simulink model "Senorless"  (R2023a)
settings: Solver=FixedStepDiscrete  StartTime=0.0  StopTime=2  FixedStep=1/FOC_FRQ  RelTol=1e-3
values from neighbouring files (symbols this model uses):
  ADC_REF = 3.6    [Senorless.sldd]
  ADC_SAMPLE_MAX = 32767.0    [Senorless.sldd]
  AMP_GAIN = 32.0    [Senorless.sldd]
  CURR_INPUT = 3276.0    [Senorless.sldd]
  CURR_KI = 380.0    [Senorless.sldd]
  CURR_KP = 0.04    [Senorless.sldd]
  CURR_LIMIT = 1.1    [Senorless.sldd]
  CURR_OVER = 34.0    [Senorless.sldd]
  CURR_POINT_GAIN = 7.0    [Senorless.sldd]
  CURR_STEP = 32760.0    [Senorless.sldd]
  CURR_UNDER = 0.03    [Senorless.sldd]
  CURR_WIDTH = 250.0    [Senorless.sldd]
  FOC_FRQ = 36000.0    [Senorless.sldd]
  GAMMA = 32767.0    [Senorless.sldd]
  HFI_ID = 2.125    [Senorless.sldd]
  IMAX = 34.0    [Senorless.sldd]
  LPF_FRQ = 300.0    [Senorless.sldd]
  MOTOR_DAMPER = 8.3E-7    [Senorless.sldd]
  MOTOR_FLUX = 0.0012713112    [Senorless.sldd]
  MOTOR_INERTIA = 1.02E-6    [Senorless.sldd]
  MOTOR_LS = 1.8E-5    [Senorless.sldd]
  MOTOR_PN = 7.0    [Senorless.sldd]
  MOTOR_RS = 0.065    [Senorless.sldd]
  NS_COMP_UD = 0.531    [Senorless.sldd]
  PLL_LIMIT = 0.95    [Senorless.sldd]
  PLL_WIDTH = 500.0    [Senorless.sldd]
  PWM_FRQ = 96000000.0    [Senorless.sldd]
  RS_HUNT = 0.002    [Senorless.sldd]
  SMOK_FRQ = 1200.0    [Senorless.sldd]
  SPD_LIMIT = 0.8    [Senorless.sldd]
  SPD_LPF_LEVEL = 15.0    [Senorless.sldd]
  SPD_MAX = 8100.0    [Senorless.sldd]
  SPD_MIN = -8100.0    [Senorless.sldd]
  SPD_REDUCE = 380.0    [Senorless.sldd]
  SPD_STEP = 3.0    [Senorless.sldd]
  SPD_WIDTH = 10.0    [Senorless.sldd]
  TS_POINT_GAIN = 10.0    [Senorless.sldd]
  UDC = 17.0    [Senorless.sldd]
  UDC_GAIN = 21.0    [Senorless.sldd]
  UDC_POINT_GAIN = 10.0    [Senorless.sldd]
undefined symbols (not defined in the file or in its folder): curr_q_ki, curr_q_kp, DiscIntNeverNeededParam, magnitude, PLL_LPF_LEVEL, Udc
libraries: simulink x20, slpidlib x5, mcbcontrolslib x4, mcbplantlib x1, autolibpmsminterior x1, autolibpmsmexterior x1, spspowerguiLib x1
(part 6 of 7)

== system Senorless/FOC_PointModel/Observers/SMO/SMO_LPF1 ==
  note: y(n)=ax(n)+(1−a)y(n−1)
  note: a =(ω c​ T s​ )/(1+ω c​ T s​ )
  input : Inport
  Constant5 : Constant  Value=32767  OutDataTypeStr=int16
  Data Store Read1 : DataStoreRead  DataStoreName=LPF_FRQ_Point  IndexOptions=Index vector (dialog)  Indices=1  OutputSizes=1
  Data Store Read7 : DataStoreRead  DataStoreName=LPF_FRQ_Point  IndexOptions=Index vector (dialog)  Indices=1  OutputSizes=1
  Product1 : Product  OutDataTypeStr=int32  RndMeth=Zero
  Product10 : Product  OutDataTypeStr=int32
  Product11 : Product  OutDataTypeStr=int32  RndMeth=Zero
  Shift Arithmetic2 : ArithShift  BitShiftNumber=15
  Shift Arithmetic3 : ArithShift  BitShiftNumber=15
  Shift Arithmetic4 : ArithShift  BitShiftNumber=4
  Sum1 : Sum  Inputs=-+  OutDataTypeStr=int32  RndMeth=Zero
  Sum10 : Sum  Inputs=-+  OutDataTypeStr=int16  RndMeth=Zero
  Sum11 : Sum  OutDataTypeStr=int32  RndMeth=Zero
  Sum2 : Sum  OutDataTypeStr=int32  RndMeth=Zero
  Unit Delay1 : UnitDelay  SampleTime=-1  HasFrameUpgradeWarning=on
  Unit Delay9 : UnitDelay  SampleTime=-1  HasFrameUpgradeWarning=on
  input1 : InportShadow
  output : Outport
  wires:
  Product10/1 -> Shift Arithmetic3/1
  Product11/1 -> Shift Arithmetic2/1
  Unit Delay9/1 -> Product10/2
  Sum10/1 -> Product10/1
  input/1 -> Product11/1
  Data Store Read7/1 -> Sum10/1, Product11/2
  Sum11/1 -> Unit Delay9/1
  Shift Arithmetic2/1 -> Sum11/1
  Shift Arithmetic3/1 -> Sum11/2
  input1/1 -> Sum1/2
  Unit Delay1/1 -> Sum2/1, Sum1/1
  Sum2/1 -> output/1, Unit Delay1/1
  Sum1/1 -> Product1/1
  Data Store Read1/1 -> Product1/2
  Product1/1 -> Shift Arithmetic4/1
  Shift Arithmetic4/1 -> Sum2/2
  Constant5/1 -> Sum10/2

== system Senorless/FOC_PointModel/Observers/SMO/SMO_LPF2 ==
  note: a =(ω c​ T s​ )/(1+ω c​ T s​ )
  note: y(n)=ax(n)+(1−a)y(n−1)
  input : Inport
  Constant5 : Constant  Value=32767  OutDataTypeStr=int16
  Data Store Read1 : DataStoreRead  DataStoreName=LPF_FRQ_Point  IndexOptions=Index vector (dialog)  Indices=1  OutputSizes=1
  Data Store Read7 : DataStoreRead  DataStoreName=LPF_FRQ_Point  IndexOptions=Index vector (dialog)  Indices=1  OutputSizes=1
  Product1 : Product  OutDataTypeStr=int32  RndMeth=Zero
  Product10 : Product  OutDataTypeStr=int32
  Product11 : Product  OutDataTypeStr=int32  RndMeth=Zero
  Shift Arithmetic2 : ArithShift  BitShiftNumber=15
  Shift Arithmetic3 : ArithShift  BitShiftNumber=15
  Shift Arithmetic4 : ArithShift  BitShiftNumber=4
  Sum1 : Sum  Inputs=-+  OutDataTypeStr=int32  RndMeth=Zero
  Sum10 : Sum  Inputs=-+  OutDataTypeStr=int16  RndMeth=Zero
  Sum11 : Sum  OutDataTypeStr=int32  RndMeth=Zero
  Sum2 : Sum  OutDataTypeStr=int32  RndMeth=Zero
  Unit Delay1 : UnitDelay  SampleTime=-1  HasFrameUpgradeWarning=on
  Unit Delay9 : UnitDelay  SampleTime=-1  HasFrameUpgradeWarning=on
  input1 : InportShadow
  output : Outport
  wires:
  Shift Arithmetic4/1 -> Sum2/2
  Product1/1 -> Shift Arithmetic4/1
  Data Store Read1/1 -> Product1/2
  Sum1/1 -> Product1/1
  Sum2/1 -> output/1, Unit Delay1/1
  Unit Delay1/1 -> Sum1/1, Sum2/1
  input1/1 -> Sum1/2
  Shift Arithmetic3/1 -> Sum11/2
  Shift Arithmetic2/1 -> Sum11/1
  Data Store Read7/1 -> Product11/2, Sum10/1
  Constant5/1 -> Sum10/2
  input/1 -> Product11/1
  Sum10/1 -> Product10/1
  Unit Delay9/1 -> Product10/2
  Product11/1 -> Shift Arithmetic2/1
  Product10/1 -> Shift Arithmetic3/1
  Sum11/1 -> Unit Delay9/1

== system Senorless/FOC_PointModel/Observers/SMO/SMO_LPF4 ==
  note: a =(ω c​ T s​ )/(1+ω c​ T s​ )
  note: y(n)=ax(n)+(1−a)y(n−1)
  input : Inport
  Constant5 : Constant  OutDataTypeStr=int16
  Data Store Read7 : DataStoreRead  DataStoreName=LPF_FRQ_Point  IndexOptions=Index vector (dialog)  Indices=1  OutputSizes=1
  Data Type Conversion6 : DataTypeConversion  OutDataTypeStr=int16  SaturateOnIntegerOverflow=off
  Product10 : Product  OutDataTypeStr=int32
  Product11 : Product  OutDataTypeStr=int32  RndMeth=Zero
  Shift Arithmetic1 : ArithShift  BitShiftNumber=-4
  Shift Arithmetic9 : ArithShift  BitShiftNumber=4
  Sum10 : Sum  Inputs=-+
  Sum11 : Sum  OutDataTypeStr=int32  RndMeth=Zero
  Unit Delay9 : UnitDelay  SampleTime=-1  HasFrameUpgradeWarning=on
  output : Outport
  wires:
  Constant5/1 -> Shift Arithmetic1/1
  Sum11/1 -> Shift Arithmetic9/1
  Data Type Conversion6/1 -> output/1, Unit Delay9/1
  Shift Arithmetic9/1 -> Data Type Conversion6/1
  Data Store Read7/1 -> Product11/2, Sum10/1
  Shift Arithmetic1/1 -> Sum10/2
  input/1 -> Product11/1
  Sum10/1 -> Product10/1
  Unit Delay9/1 -> Product10/2
  Product11/1 -> Sum11/1
  Product10/1 -> Sum11/2

== system Senorless/FOC_PointModel/Observers/SMO/SMO_LPF5 ==
  note: y(n)=ax(n)+(1−a)y(n−1)
  note: a =(ω c​ T s​ )/(1+ω c​ T s​ )
  input : Inport
  Constant5 : Constant  OutDataTypeStr=int16
  Data Store Read7 : DataStoreRead  DataStoreName=LPF_FRQ_Point  IndexOptions=Index vector (dialog)  Indices=1  OutputSizes=1
  Data Type Conversion6 : DataTypeConversion  OutDataTypeStr=int16  SaturateOnIntegerOverflow=off
  Product10 : Product  OutDataTypeStr=int32
  Product11 : Product  OutDataTypeStr=int32  RndMeth=Zero
  Shift Arithmetic1 : ArithShift  BitShiftNumber=-4
  Shift Arithmetic9 : ArithShift  BitShiftNumber=4
  Sum10 : Sum  Inputs=-+
  Sum11 : Sum  OutDataTypeStr=int32  RndMeth=Zero
  Unit Delay9 : UnitDelay  SampleTime=-1  HasFrameUpgradeWarning=on
  output : Outport
  wires:
  Product10/1 -> Sum11/2
  Product11/1 -> Sum11/1
  Unit Delay9/1 -> Product10/2
  Sum10/1 -> Product10/1
  input/1 -> Product11/1
  Shift Arithmetic1/1 -> Sum10/2
  Data Store Read7/1 -> Sum10/1, Product11/2
  Shift Arithmetic9/1 -> Data Type Conversion6/1
  Data Type Conversion6/1 -> Unit Delay9/1, output/1
  Sum11/1 -> Shift Arithmetic9/1
  Constant5/1 -> Shift Arithmetic1/1

== system Senorless/FOC_PointModel/Observers/SMO/Subsystem ==
  ialpha_err : Inport
  ialpha_hat : Inport  Port=2
  ibeta_hat : Inport  Port=3
  ibeta_err : Inport  Port=4
  Constant : Constant  Value=MOTOR_RS
  Display : Display
  Display1 : Display
  Divide : Product  Inputs=*/
  Gain4 : Gain  Gain=1/MOTOR_LS/FOC_FRQ
  Product : Product
  Product1 : Product
  Scope : Scope
  Scope1 : Scope  NumInputPorts=2
  Scope2 : Scope
  Scope3 : Scope  NumInputPorts=2
  Sum : Sum  Inputs=|++
  Sum2 : Sum
  Unit Delay : UnitDelay  SampleTime=-1  HasFrameUpgradeWarning=on
  Output : Outport
  wires:
  ibeta_hat/1 -> Product1/2
  ialpha_hat/1 -> Scope3/2, Product/2
  Product/1 -> Scope1/1, Sum2/1
  Constant/1 -> Divide/1, Display/1
  Divide/1 -> Display1/1
  Product1/1 -> Scope1/2, Sum2/2
  ialpha_err/1 -> Scope3/1, Product/1
  ibeta_err/1 -> Product1/1
  Gain4/1 -> Sum/1
  Sum/1 -> Unit Delay/1, Output/1, Scope2/1, Divide/2
  Unit Delay/1 -> Sum/2
  Sum2/1 -> Scope/1, Gain4/1

== system Senorless/FOC_PointModel/Observers/滤波器/LPF ==
  note: a =(ω c​ T s​ )/(1+ω c​ T s​ )
  note: y(n)=ax(n)+(1−a)y(n−1)
  input : Inport
  Constant1 : Constant  Value=8  OutDataTypeStr=int16
  Constant5 : Constant  OutDataTypeStr=int16
  Product10 : Product  OutDataTypeStr=int32
  Product11 : Product  OutDataTypeStr=int32  RndMeth=Zero
  Saturation : Saturate  UpperLimit=15  LowerLimit=0  RndMeth=Zero
  Shift Arithmetic1 : ArithShift  BitShiftNumber=-4
  Shift Arithmetic9 : ArithShift  BitShiftNumber=4
  Sum10 : Sum  Inputs=-+
  Sum11 : Sum  OutDataTypeStr=int32  RndMeth=Zero
  Unit Delay9 : UnitDelay  SampleTime=-1  HasFrameUpgradeWarning=on
  output : Outport
  wires:
  Constant1/1 -> Saturation/1
  Constant5/1 -> Shift Arithmetic1/1
  Sum11/1 -> Shift Arithmetic9/1
  Shift Arithmetic9/1 -> output/1, Unit Delay9/1
  Shift Arithmetic1/1 -> Sum10/2
  Sum10/1 -> Product10/1
  Product11/1 -> Sum11/1
  Product10/1 -> Sum11/2
  Unit Delay9/1 -> Product11/1
  input/1 -> Product10/2
  Saturation/1 -> Sum10/1, Product11/2

== system Senorless/FOC_PointModel/Observers/滤波器/积分器4 ==
  input : Inport
  Constant : Constant  OutDataTypeStr=int16
  Data Store Read1 : DataStoreRead  DataStoreName=Ts_Point  IndexOptions=Index vector (dialog)  Indices=1  OutputSizes=1
  Data Type Conversion3 : DataTypeConversion  Commented=on  OutDataTypeStr=int16  SaturateOnIntegerOverflow=off
  Divide : Product  Commented=on  Inputs=*/  OutDataTypeStr=int32  RndMeth=Zero
  Product1 : Product  OutDataTypeStr=int32  RndMeth=Zero
  Product2 : Product  OutDataTypeStr=int32  RndMeth=Zero
  Shift Arithmetic : ArithShift  BitShiftNumberSource=Input port  BitShiftNumber=8  BitShiftDirection=Right
      settings: InputPortMap=u0,p1
  Sum : Sum  Inputs=|++  OutDataTypeStr=int32  RndMeth=Zero
  Ts适当放大的缩小系数， 详见初始化模块 : ArithShift  Commented=on  BitShiftNumber=TS_POINT_GAIN  DiagnosticForOORShift=Error
  Unit Delay : UnitDelay  SampleTime=-1  HasFrameUpgradeWarning=on
  周期定点化适当放大2^n : Constant  Value=TS_POINT_GAIN
  积分器运行频率 : Constant  Commented=on  Value=FOC_FRQ
  这个是缩小周期增益的 : ArithShift  BitShiftNumber=15  DiagnosticForOORShift=Error
  output : Outport
  wires:
  这个是缩小周期增益的/1 -> output/1
  Product2/1 -> Product1/2
  积分器运行频率/1 -> Data Type Conversion3/1
  Data Type Conversion3/1 -> Divide/2
  周期定点化适当放大2^n/1 -> Shift Arithmetic/2
  Sum/1 -> Unit Delay/1, 这个是缩小周期增益的/1
  Unit Delay/1 -> Sum/2
  input/1 -> Shift Arithmetic/1
  Shift Arithmetic/1 -> Product2/2
  Data Store Read1/1 -> Product2/1
  Constant/1 -> Product1/1
  Product1/1 -> Sum/1

== system Senorless/FOC_PointModel/Observers/滤波器/积分器5 ==
  input : Inport
  Constant : Constant  OutDataTypeStr=int16
  Data Store Read1 : DataStoreRead  DataStoreName=Ts_Point  IndexOptions=Index vector (dialog)  Indices=1  OutputSizes=1
  Data Type Conversion3 : DataTypeConversion  Commented=on  OutDataTypeStr=int16  SaturateOnIntegerOverflow=off
  Divide : Product  Commented=on  Inputs=*/  OutDataTypeStr=int32  RndMeth=Zero
  Product1 : Product  OutDataTypeStr=int32  RndMeth=Zero
  Product2 : Product  OutDataTypeStr=int32  RndMeth=Zero
  Shift Arithmetic : ArithShift  BitShiftNumberSource=Input port  BitShiftNumber=8  BitShiftDirection=Right
      settings: InputPortMap=u0,p1
  Sum : Sum  Inputs=|++  OutDataTypeStr=int32  RndMeth=Zero
  Ts适当放大的缩小系数， 详见初始化模块 : ArithShift  Commented=on  BitShiftNumber=TS_POINT_GAIN  DiagnosticForOORShift=Error
  Unit Delay : UnitDelay  SampleTime=-1  HasFrameUpgradeWarning=on
  周期定点化适当放大2^n : Constant  Value=TS_POINT_GAIN
  积分器运行频率 : Constant  Commented=on  Value=FOC_FRQ
  这个是缩小周期增益的 : ArithShift  BitShiftNumber=15  DiagnosticForOORShift=Error
  output : Outport
  wires:
  这个是缩小周期增益的/1 -> output/1
  Product2/1 -> Product1/2
  积分器运行频率/1 -> Data Type Conversion3/1
  Data Type Conversion3/1 -> Divide/2
  周期定点化适当放大2^n/1 -> Shift Arithmetic/2
  Sum/1 -> Unit Delay/1, 这个是缩小周期增益的/1
  Unit Delay/1 -> Sum/2
  input/1 -> Shift Arithmetic/1
  Shift Arithmetic/1 -> Product2/2
  Data Store Read1/1 -> Product2/1
  Constant/1 -> Product1/1
  Product1/1 -> Sum/1

== system Senorless/FOC_PointModel/Observers/纯浮点NFO/LPF ==
  note: a =(ω c​ T s​ )/(1+ω c​ T s​ )
  note: y(n)=ax(n)+(1−a)y(n−1)
  input : Inport
  Constant1 : Constant  Value=SPD_LPF_LEVEL  OutDataTypeStr=int16
  Constant5 : Constant  OutDataTypeStr=int16
  Product10 : Product  OutDataTypeStr=int32
  Product11 : Product  OutDataTypeStr=int32  RndMeth=Zero
  Saturation : Saturate  UpperLimit=15  LowerLimit=0  RndMeth=Zero
  Shift Arithmetic1 : ArithShift  BitShiftNumber=-4
  Shift Arithmetic9 : ArithShift  BitShiftNumber=4
  Sum10 : Sum  Inputs=-+
  Sum11 : Sum  OutDataTypeStr=int32  RndMeth=Zero
  Unit Delay9 : UnitDelay  SampleTime=-1  HasFrameUpgradeWarning=on
  output : Outport
  wires:
  Constant1/1 -> Saturation/1
  Constant5/1 -> Shift Arithmetic1/1
  Sum11/1 -> Shift Arithmetic9/1
  Shift Arithmetic9/1 -> output/1, Unit Delay9/1
  Shift Arithmetic1/1 -> Sum10/2
  Sum10/1 -> Product10/1
  Product11/1 -> Sum11/1
  Product10/1 -> Sum11/2
  Unit Delay9/1 -> Product11/1
  input/1 -> Product10/2
  Saturation/1 -> Sum10/1, Product11/2

== system Senorless/FOC_PointModel/Park/滤波器/积分器4 ==
  input : Inport
  Constant : Constant  OutDataTypeStr=int16
  Data Store Read1 : DataStoreRead  DataStoreName=Ts_Point  IndexOptions=Index vector (dialog)  Indices=1  OutputSizes=1
  Data Type Conversion3 : DataTypeConversion  Commented=on  OutDataTypeStr=int16  SaturateOnIntegerOverflow=off
  Divide : Product  Commented=on  Inputs=*/  OutDataTypeStr=int32  RndMeth=Zero
  Product1 : Product  OutDataTypeStr=int32  RndMeth=Zero
  Product2 : Product  OutDataTypeStr=int32  RndMeth=Zero
  Shift Arithmetic : ArithShift  BitShiftNumberSource=Input port  BitShiftNumber=8  BitShiftDirection=Right
      settings: InputPortMap=u0,p1
  Sum : Sum  Inputs=|++  OutDataTypeStr=int32  RndMeth=Zero
  Ts适当放大的缩小系数， 详见初始化模块 : ArithShift  Commented=on  BitShiftNumber=TS_POINT_GAIN  DiagnosticForOORShift=Error
  Unit Delay : UnitDelay  SampleTime=-1  HasFrameUpgradeWarning=on
  周期定点化适当放大2^n : Constant  Value=TS_POINT_GAIN
  积分器运行频率 : Constant  Commented=on  Value=FOC_FRQ
  这个是缩小周期增益的 : ArithShift  BitShiftNumber=15  DiagnosticForOORShift=Error
  output : Outport
  wires:
  这个是缩小周期增益的/1 -> output/1
  Product2/1 -> Product1/2
  积分器运行频率/1 -> Data Type Conversion3/1
  Data Type Conversion3/1 -> Divide/2
  周期定点化适当放大2^n/1 -> Shift Arithmetic/2
  Sum/1 -> Unit Delay/1, 这个是缩小周期增益的/1
  Unit Delay/1 -> Sum/2
  input/1 -> Shift Arithmetic/1
  Shift Arithmetic/1 -> Product2/2
  Data Store Read1/1 -> Product2/1
  Constant/1 -> Product1/1
  Product1/1 -> Sum/1

== system Senorless/FOC_PointModel/Park/滤波器/积分器5 ==
  input : Inport
  Constant : Constant  OutDataTypeStr=int16
  Data Store Read1 : DataStoreRead  DataStoreName=Ts_Point  IndexOptions=Index vector (dialog)  Indices=1  OutputSizes=1
  Data Type Conversion3 : DataTypeConversion  Commented=on  OutDataTypeStr=int16  SaturateOnIntegerOverflow=off
  Divide : Product  Commented=on  Inputs=*/  OutDataTypeStr=int32  RndMeth=Zero
  Product1 : Product  OutDataTypeStr=int32  RndMeth=Zero
  Product2 : Product  OutDataTypeStr=int32  RndMeth=Zero
  Shift Arithmetic : ArithShift  BitShiftNumberSource=Input port  BitShiftNumber=8  BitShiftDirection=Right
      settings: InputPortMap=u0,p1
  Sum : Sum  Inputs=|++  OutDataTypeStr=int32  RndMeth=Zero
  Ts适当放大的缩小系数， 详见初始化模块 : ArithShift  Commented=on  BitShiftNumber=TS_POINT_GAIN  DiagnosticForOORShift=Error
  Unit Delay : UnitDelay  SampleTime=-1  HasFrameUpgradeWarning=on
  周期定点化适当放大2^n : Constant  Value=TS_POINT_GAIN
  积分器运行频率 : Constant  Commented=on  Value=FOC_FRQ
  这个是缩小周期增益的 : ArithShift  BitShiftNumber=15  DiagnosticForOORShift=Error
  output : Outport
  wires:
  这个是缩小周期增益的/1 -> output/1
  Product2/1 -> Product1/2
  积分器运行频率/1 -> Data Type Conversion3/1
  Data Type Conversion3/1 -> Divide/2
  周期定点化适当放大2^n/1 -> Shift Arithmetic/2
  Sum/1 -> Unit Delay/1, 这个是缩小周期增益的/1
  Unit Delay/1 -> Sum/2
  input/1 -> Shift Arithmetic/1
  Shift Arithmetic/1 -> Product2/2
  Data Store Read1/1 -> Product2/1
  Constant/1 -> Product1/1
  Product1/1 -> Sum/1

== system Senorless/FOC_PointModel/idq_Controller/PI Controller/积分器 ==
  Ki : Inport
  input : Inport  Port=2
  Constant : Constant  Value=32767*32767  OutDataTypeStr=int32
  Data Store Read1 : DataStoreRead  DataStoreName=Ts_Point  IndexOptions=Index vector (dialog)  Indices=1  OutputSizes=1
  Data Store Read3 : DataStoreRead  DataStoreName=Curr_Limit  IndexOptions=Index vector (dialog)  Indices=1  OutputSizes=1
  Data Type Conversion3 : DataTypeConversion  Commented=on  OutDataTypeStr=int16  SaturateOnIntegerOverflow=off
  Divide : Product  Commented=on  Inputs=*/  OutDataTypeStr=int32  RndMeth=Zero
  Gain : Gain  Gain=-1  OutDataTypeStr=int32  RndMeth=Zero
  Product1 : Product  OutDataTypeStr=int32  RndMeth=Zero
  Product2 : Product  OutDataTypeStr=int32  RndMeth=Zero
  Saturation Dynamic2 : simulink/Discontinuities/Saturation Dynamic  OutMin=[]  OutMax=[]  OutDataTypeStr=Inherit: Same as second input  OutDataType=fixdt(1, 16)  OutScaling=2^-10  RndMeth=Zero  DoSatur=off
  Shift Arithmetic : ArithShift  BitShiftNumberSource=Input port  BitShiftNumber=8  BitShiftDirection=Right
      settings: InputPortMap=u0,p1
  Sum : Sum  Inputs=|++  OutDataTypeStr=int32  RndMeth=Zero
  Sum2 : Sum  Inputs=-+  OutDataTypeStr=int32  RndMeth=Zero
  Ts适当放大的缩小系数， 详见初始化模块 : ArithShift  Commented=on  BitShiftNumber=TS_POINT_GAIN  DiagnosticForOORShift=Error
  Unit Delay : UnitDelay  SampleTime=-1  HasFrameUpgradeWarning=on
  周期定点化适当放大2^n : Constant  Value=TS_POINT_GAIN
  积分器运行频率 : Constant  Commented=on  Value=FOC_FRQ
  这个是缩小周期增益的 : ArithShift  BitShiftNumber=15  DiagnosticForOORShift=Error
  output : Outport
  wires:
  积分器运行频率/1 -> Data Type Conversion3/1
  Data Type Conversion3/1 -> Divide/2
  Product2/1 -> 这个是缩小周期增益的/1
  Ki/1 -> Shift Arithmetic/1
  Shift Arithmetic/1 -> Product1/1
  Data Store Read1/1 -> Product2/1
  input/1 -> Product2/2
  周期定点化适当放大2^n/1 -> Shift Arithmetic/2
  Constant/1 -> Sum2/2
  Data Store Read3/1 -> Sum2/1, [limit]
  Sum2/1 -> [Limit1]
  [limit] -> Gain/1
  Product1/1 -> Sum/1
  这个是缩小周期增益的/1 -> Product1/2
  Unit Delay/1 -> Sum/2
  Gain/1 -> Saturation Dynamic2/3
  Sum/1 -> Saturation Dynamic2/2
  [limit] -> Saturation Dynamic2/1
  Saturation Dynamic2/1 -> Unit Delay/1, output/1

== system Senorless/FOC_PointModel/idq_Controller/PI Controller1/积分器 ==
  Ki : Inport
  input : Inport  Port=2
  Constant : Constant  Value=32767*32767  OutDataTypeStr=int32
  Data Store Read1 : DataStoreRead  DataStoreName=Ts_Point  IndexOptions=Index vector (dialog)  Indices=1  OutputSizes=1
  Data Store Read3 : DataStoreRead  DataStoreName=Curr_Limit  IndexOptions=Index vector (dialog)  Indices=1  OutputSizes=1
  Data Type Conversion3 : DataTypeConversion  Commented=on  OutDataTypeStr=int16  SaturateOnIntegerOverflow=off
  Divide : Product  Commented=on  Inputs=*/  OutDataTypeStr=int32  RndMeth=Zero
  Gain : Gain  Gain=-1  OutDataTypeStr=int32  RndMeth=Zero
  Product1 : Product  OutDataTypeStr=int32  RndMeth=Zero
  Product2 : Product  OutDataTypeStr=int32  RndMeth=Zero
  Saturation Dynamic2 : simulink/Discontinuities/Saturation Dynamic  OutMin=[]  OutMax=[]  OutDataTypeStr=Inherit: Same as second input  OutDataType=fixdt(1, 16)  OutScaling=2^-10  RndMeth=Zero  DoSatur=off
  Scope : Scope
  Shift Arithmetic : ArithShift  BitShiftNumberSource=Input port  BitShiftNumber=8  BitShiftDirection=Right
      settings: InputPortMap=u0,p1
  Sum : Sum  Inputs=|++  OutDataTypeStr=int32  RndMeth=Zero
  Sum2 : Sum  Inputs=-+  OutDataTypeStr=int32  RndMeth=Zero
  Ts适当放大的缩小系数， 详见初始化模块 : ArithShift  Commented=on  BitShiftNumber=TS_POINT_GAIN  DiagnosticForOORShift=Error
  Unit Delay : UnitDelay  SampleTime=-1  HasFrameUpgradeWarning=on
  周期定点化适当放大2^n : Constant  Value=TS_POINT_GAIN
  积分器运行频率 : Constant  Commented=on  Value=FOC_FRQ
  这个是缩小周期增益的 : ArithShift  BitShiftNumber=15  DiagnosticForOORShift=Error
  output : Outport
  wires:
  Saturation Dynamic2/1 -> Unit Delay/1, output/1
  [limit] -> Saturation Dynamic2/1
  Sum/1 -> Saturation Dynamic2/2
  Gain/1 -> Saturation Dynamic2/3
  Unit Delay/1 -> Sum/2
  这个是缩小周期增益的/1 -> Product1/2
  Product1/1 -> Scope/1, Sum/1
  [limit] -> Gain/1
  Sum2/1 -> [Limit1]
  Data Store Read3/1 -> [limit], Sum2/1
  Constant/1 -> Sum2/2
  周期定点化适当放大2^n/1 -> Shift Arithmetic/2
  input/1 -> Product2/2
  Data Store Read1/1 -> Product2/1
  Shift Arithmetic/1 -> Product1/1
  Ki/1 -> Shift Arithmetic/1
  Product2/1 -> 这个是缩小周期增益的/1
  Data Type Conversion3/1 -> Divide/2
  积分器运行频率/1 -> Data Type Conversion3/1

== system Senorless/FOC_PointModel/idq_Controller/PI Controller2/积分器//双边沿初始化 ==
  Ki : Inport
  input : Inport  Port=2
  Xo : Inport  Port=3
  Reset : Inport  Port=4
  Constant : Constant  Value=32767*32767  OutDataTypeStr=int32
  Data Store Memory : DataStoreMemory  DataStoreName=tmp  WriteAfterWriteMsg=warning  ShowAdditionalParam=off  OutDataTypeStr=int32
  Data Store Read : DataStoreRead  DataStoreName=tmp  IndexOptions=Index vector (dialog)  Indices=1  OutputSizes=1
  Data Store Read1 : DataStoreRead  DataStoreName=Ts_Point  IndexOptions=Index vector (dialog)  Indices=1  OutputSizes=1
  Data Store Read3 : DataStoreRead  DataStoreName=Curr_Limit  IndexOptions=Index vector (dialog)  Indices=1  OutputSizes=1
  Data Store Write : DataStoreWrite  DataStoreName=tmp  IndexOptions=Index vector (dialog)  Indices=1  OutputSizes=1
  Data Type Conversion : DataTypeConversion  OutDataTypeStr=int16  SaturateOnIntegerOverflow=off
  Data Type Conversion2 : DataTypeConversion  OutDataTypeStr=int32  SaturateOnIntegerOverflow=off
  Data Type Conversion3 : DataTypeConversion  Commented=on  OutDataTypeStr=int16  SaturateOnIntegerOverflow=off
  Divide : Product  Commented=on  Inputs=*/  OutDataTypeStr=int32  RndMeth=Zero
  Gain : Gain  Gain=-1  OutDataTypeStr=int32  RndMeth=Zero
  Gain1 : Gain  Gain=-1  OutDataTypeStr=int32  RndMeth=Zero
  MATLAB Function : MATLAB Function  TreatAsAtomicUnit=on
  MATLAB Function1 : MATLAB Function  TreatAsAtomicUnit=on
  MATLAB Function2 : MATLAB Function  TreatAsAtomicUnit=on
  Product1 : Product  OutDataTypeStr=int32  RndMeth=Zero
  Product2 : Product  OutDataTypeStr=int32  RndMeth=Zero
  Reset_Block : Subsystem
  Scope : Scope  NumInputPorts=2
  Sum : Sum  Inputs=|++  OutDataTypeStr=int32  RndMeth=Zero
  Sum1 : Sum  Inputs=|+-  OutDataTypeStr=int32  RndMeth=Zero
  Sum2 : Sum  Inputs=-+  OutDataTypeStr=int32  RndMeth=Zero
  Ts适当放大的缩小系数， 详见初始化模块 : ArithShift  Commented=on  BitShiftNumber=TS_POINT_GAIN  DiagnosticForOORShift=Error
  Unit Delay : UnitDelay  SampleTime=-1  HasFrameUpgradeWarning=on
  周期定点化适当放大2^n : Constant  Value=TS_POINT_GAIN
  积分器运行频率 : Constant  Commented=on  Value=FOC_FRQ
  这个是缩小周期增益的 : ArithShift  BitShiftNumber=15  DiagnosticForOORShift=Error
  output : Outport
  wires:
  Data Type Conversion/1 -> Product1/2
  MATLAB Function1/1(out) -> Sum/1, Sum1/2, Scope/2
  [Limit1] -> MATLAB Function1/2(up), Gain1/1
  Gain1/1 -> MATLAB Function1/3(low)
  [limit] -> MATLAB Function/2(up), Gain/1
  Gain/1 -> MATLAB Function/3(low)
  Sum2/1 -> [Limit1]
  Data Store Read3/1 -> [limit], Sum2/1
  Constant/1 -> Sum2/2
  周期定点化适当放大2^n/1 -> MATLAB Function2/2(n)
  input/1 -> Product2/2
  Data Store Read1/1 -> Product2/1
  Sum1/1 -> Reset_Block/1(Xo)
  Data Type Conversion2/1 -> Sum1/1
  Product1/1 -> MATLAB Function1/1(in), Scope/1
  Sum/1 -> MATLAB Function/1(in)
  MATLAB Function2/1(out) -> Product1/1
  Reset/1 -> Reset_Block/Trigger
  Ki/1 -> MATLAB Function2/1(in)
  这个是缩小周期增益的/1 -> Data Type Conversion/1
  Product2/1 -> 这个是缩小周期增益的/1
  Data Type Conversion3/1 -> Divide/2
  Xo/1 -> Data Type Conversion2/1
  积分器运行频率/1 -> Data Type Conversion3/1
  Unit Delay/1 -> Data Store Write/1
  Data Store Read/1 -> Sum/2
  MATLAB Function/1(out) -> Unit Delay/1, output/1

== system Senorless/FOC_PointModel/观测器闭环//速度环/PI Controller/积分器1 ==
  note: 速度环积分int64为了提高低速时精度，int64使用需慎重
  Ki : Inport
  input : Inport  Port=2
  init : Inport  Port=3
  Constant : Constant  OutDataTypeStr=int64
  Constant1 : Constant  Value=32767  OutDataTypeStr=int32
  Data Store Read1 : DataStoreRead  DataStoreName=Ts_Point  IndexOptions=Index vector (dialog)  Indices=1  OutputSizes=1
  Data Store Read2 : DataStoreRead  DataStoreName=Speed_Limit  IndexOptions=Index vector (dialog)  Indices=1  OutputSizes=1
  Data Type Conversion : DataTypeConversion  OutDataTypeStr=int64  SaturateOnIntegerOverflow=off  RndMeth=Floor
  Data Type Conversion1 : DataTypeConversion  OutDataTypeStr=int32  SaturateOnIntegerOverflow=off
  Data Type Conversion2 : DataTypeConversion  OutDataTypeStr=int64  SaturateOnIntegerOverflow=off
  Data Type Conversion3 : DataTypeConversion  Commented=on  OutDataTypeStr=int16  SaturateOnIntegerOverflow=off
  Delay : Delay  DelayLength=1  InitialConditionSource=Input port
      settings: InputPortMap=u0,p4
  Divide : Product  Commented=on  Inputs=*/  OutDataTypeStr=int32  RndMeth=Zero
  Gain : Gain  Gain=-1  RndMeth=Zero  OutDataTypeStr=Inherit: Same as input
  Product1 : Product  OutDataTypeStr=int32  RndMeth=Zero
  Product2 : Product  OutDataTypeStr=int32  RndMeth=Zero
  Saturation Dynamic2 : simulink/Discontinuities/Saturation Dynamic  OutMin=[]  OutMax=[]  OutDataTypeStr=Inherit: Same as second input  OutDataType=fixdt(1, 16)  OutScaling=2^-10  RndMeth=Zero  DoSatur=off
  Scope : Scope
  Shift Arithmetic : ArithShift  BitShiftNumberSource=Input port  BitShiftNumber=8  BitShiftDirection=Right
      settings: InputPortMap=u0,p1
  Shift Arithmetic1 : ArithShift  BitShiftNumberSource=Input port  BitShiftNumber=8  BitShiftDirection=Left
      settings: InputPortMap=u0,p1
  Shift Arithmetic2 : ArithShift  BitShiftNumber=-15
  Shift Arithmetic3 : ArithShift  BitShiftNumberSource=Input port  BitShiftNumber=8  BitShiftDirection=Left
      settings: InputPortMap=u0,p1
  Sum : Sum  Inputs=|++  OutDataTypeStr=int64  RndMeth=Zero
  Sum1 : Sum  Inputs=-+  OutDataTypeStr=int32  RndMeth=Zero
  Ts适当放大的缩小系数， 详见初始化模块 : ArithShift  Commented=on  BitShiftNumber=TS_POINT_GAIN  DiagnosticForOORShift=Error
  Unit Delay : UnitDelay  SampleTime=-1  HasFrameUpgradeWarning=on
  周期定点化适当放大2^n : Constant  Value=TS_POINT_GAIN
  周期定点化适当放大2^n1 : Constant  Value=TS_POINT_GAIN
  周期定点化适当放大2^n2 : Constant  Value=TS_POINT_GAIN
  积分器运行频率 : Constant  Commented=on  Value=FOC_FRQ
  这个是缩小周期增益的 : ArithShift  BitShiftNumber=15  DiagnosticForOORShift=Error
  这个是缩小周期增益的1 : ArithShift  BitShiftNumber=-15  DiagnosticForOORShift=Error
  output : Outport
  wires:
  [limit] -> Gain/1, Saturation Dynamic2/1
  Sum/1 -> Saturation Dynamic2/2
  Gain/1 -> Saturation Dynamic2/3
  Delay/1 -> Sum/2
  input/1 -> Product2/2
  Data Store Read1/1 -> Product2/1
  Data Type Conversion3/1 -> Divide/2
  积分器运行频率/1 -> Data Type Conversion3/1
  Data Store Read2/1 -> Data Type Conversion/1, Sum1/1
  Constant1/1 -> Sum1/2
  Sum1/1 -> [Limit1]
  周期定点化适当放大2^n/1 -> Shift Arithmetic/2
  Saturation Dynamic2/1 -> Delay/1, Scope/1, 这个是缩小周期增益的/1
  Product2/1 -> Product1/2
  Ki/1 -> Product1/1
  Shift Arithmetic/1 -> Data Type Conversion1/1
  Shift Arithmetic1/1 -> [limit]
  周期定点化适当放大2^n1/1 -> Shift Arithmetic1/2
  Product1/1 -> Sum/1
  这个是缩小周期增益的/1 -> Shift Arithmetic/1
  Shift Arithmetic2/1 -> Shift Arithmetic1/1
  Data Type Conversion/1 -> Shift Arithmetic2/1
  Data Type Conversion1/1 -> output/1
  init/1 -> Data Type Conversion2/1
  周期定点化适当放大2^n2/1 -> Shift Arithmetic3/2
  这个是缩小周期增益的1/1 -> Delay/2
  Shift Arithmetic3/1 -> 这个是缩小周期增益的1/1
  Data Type Conversion2/1 -> Shift Arithmetic3/1

== system Senorless/FOC_PointModel/NS辨识/加速积分角度/积分器/Reset_Block ==
  Xo : Inport
  Trigger : TriggerPort  VariantControl=(inherit)  OutputDataType=int8  InitialTriggerSignalState=zero  PortDimensions=1
  Data Store Write1 : DataStoreWrite  DataStoreName=tmp  IndexOptions=Index vector (dialog)  Indices=1  OutputSizes=1
  wires:
  Xo/1 -> Data Store Write1/1

== system Senorless/FOC_PointModel/NS辨识/加速积分角度/积分器2/Reset_Block ==
  Xo : Inport
  Trigger : TriggerPort  VariantControl=(inherit)  OutputDataType=int8  InitialTriggerSignalState=zero  PortDimensions=1
  Data Store Write1 : DataStoreWrite  DataStoreName=tmp  IndexOptions=Index vector (dialog)  Indices=1  OutputSizes=1
  wires:
  Xo/1 -> Data Store Write1/1

== system Senorless/FOC_PointModel/Observers/PLL/PI Controller/积分器 ==
  Ki : Inport
  input : Inport  Port=2
  Constant : Constant  Value=32767*32767  OutDataTypeStr=int32
  Data Store Read1 : DataStoreRead  DataStoreName=Ts_Point  IndexOptions=Index vector (dialog)  Indices=1  OutputSizes=1
  Data Store Read3 : DataStoreRead  DataStoreName=PLL_Limit  IndexOptions=Index vector (dialog)  Indices=1  OutputSizes=1
  Data Type Conversion3 : DataTypeConversion  Commented=on  OutDataTypeStr=int16  SaturateOnIntegerOverflow=off
  Divide : Product  Commented=on  Inputs=*/  OutDataTypeStr=int32  RndMeth=Zero
  Gain : Gain  Gain=-1  OutDataTypeStr=int32  RndMeth=Zero
  Product1 : Product  OutDataTypeStr=int32  RndMeth=Zero
  Product2 : Product  OutDataTypeStr=int32  RndMeth=Zero
  Saturation Dynamic2 : simulink/Discontinuities/Saturation Dynamic  OutMin=[]  OutMax=[]  OutDataTypeStr=Inherit: Same as second input  OutDataType=fixdt(1, 16)  OutScaling=2^-10  RndMeth=Zero  DoSatur=off
  Shift Arithmetic : ArithShift  BitShiftNumberSource=Input port  BitShiftNumber=8  BitShiftDirection=Right
      settings: InputPortMap=u0,p1
  Sum : Sum  Inputs=|++  OutDataTypeStr=int32  RndMeth=Zero
  Sum2 : Sum  Inputs=-+  OutDataTypeStr=int32  RndMeth=Zero
  Ts适当放大的缩小系数， 详见初始化模块 : ArithShift  Commented=on  BitShiftNumber=TS_POINT_GAIN  DiagnosticForOORShift=Error
  Unit Delay : UnitDelay  SampleTime=-1  HasFrameUpgradeWarning=on
  周期定点化适当放大2^n : Constant  Value=TS_POINT_GAIN
  积分器运行频率 : Constant  Commented=on  Value=FOC_FRQ
  这个是缩小周期增益的 : ArithShift  BitShiftNumber=15  DiagnosticForOORShift=Error
  output : Outport
  wires:
  积分器运行频率/1 -> Data Type Conversion3/1
  Data Type Conversion3/1 -> Divide/2
  Product2/1 -> 这个是缩小周期增益的/1
  Ki/1 -> Shift Arithmetic/1
  Shift Arithmetic/1 -> Product1/1
  Data Store Read1/1 -> Product2/1
  input/1 -> Product2/2
  周期定点化适当放大2^n/1 -> Shift Arithmetic/2
  [Limit] -> Gain/1
  Data Store Read3/1 -> Sum2/1, [Limit]
  Constant/1 -> Sum2/2
  Sum2/1 -> [Limit1]
  这个是缩小周期增益的/1 -> Product1/2
  Unit Delay/1 -> Sum/2
  Gain/1 -> Saturation Dynamic2/3
  Sum/1 -> Saturation Dynamic2/2
  [Limit] -> Saturation Dynamic2/1
  Saturation Dynamic2/1 -> Unit Delay/1, output/1
  Product1/1 -> Sum/1

== system Senorless/FOC_PointModel/Observers/PLL2/PI Controller/积分器 ==
  Ki : Inport
  input : Inport  Port=2
  Constant : Constant  Value=32767*32767  OutDataTypeStr=int32
  Data Store Read1 : DataStoreRead  DataStoreName=Ts_Point  IndexOptions=Index vector (dialog)  Indices=1  OutputSizes=1
  Data Store Read3 : DataStoreRead  DataStoreName=PLL_Limit  IndexOptions=Index vector (dialog)  Indices=1  OutputSizes=1
  Data Type Conversion3 : DataTypeConversion  Commented=on  OutDataTypeStr=int16  SaturateOnIntegerOverflow=off
  Divide : Product  Commented=on  Inputs=*/  OutDataTypeStr=int32  RndMeth=Zero
  Gain : Gain  Gain=-1  OutDataTypeStr=int32  RndMeth=Zero
  Product1 : Product  OutDataTypeStr=int32  RndMeth=Zero
  Product2 : Product  OutDataTypeStr=int32  RndMeth=Zero
  Saturation Dynamic2 : simulink/Discontinuities/Saturation Dynamic  OutMin=[]  OutMax=[]  OutDataTypeStr=Inherit: Same as second input  OutDataType=fixdt(1, 16)  OutScaling=2^-10  RndMeth=Zero  DoSatur=off
  Shift Arithmetic : ArithShift  BitShiftNumberSource=Input port  BitShiftNumber=8  BitShiftDirection=Right
      settings: InputPortMap=u0,p1
  Sum : Sum  Inputs=|++  OutDataTypeStr=int32  RndMeth=Zero
  Sum2 : Sum  Inputs=-+  OutDataTypeStr=int32  RndMeth=Zero
  Ts适当放大的缩小系数， 详见初始化模块 : ArithShift  Commented=on  BitShiftNumber=TS_POINT_GAIN  DiagnosticForOORShift=Error
  Unit Delay : UnitDelay  SampleTime=-1  HasFrameUpgradeWarning=on
  周期定点化适当放大2^n : Constant  Value=TS_POINT_GAIN
  积分器运行频率 : Constant  Commented=on  Value=FOC_FRQ
  这个是缩小周期增益的 : ArithShift  BitShiftNumber=15  DiagnosticForOORShift=Error
  output : Outport
  wires:
  Product1/1 -> Sum/1
  Saturation Dynamic2/1 -> output/1, Unit Delay/1
  [Limit] -> Saturation Dynamic2/1
  Sum/1 -> Saturation Dynamic2/2
  Gain/1 -> Saturation Dynamic2/3
  Unit Delay/1 -> Sum/2
  这个是缩小周期增益的/1 -> Product1/2
  Sum2/1 -> [Limit1]
  Constant/1 -> Sum2/2
  Data Store Read3/1 -> [Limit], Sum2/1
  [Limit] -> Gain/1
  周期定点化适当放大2^n/1 -> Shift Arithmetic/2
  input/1 -> Product2/2
  Data Store Read1/1 -> Product2/1
  Shift Arithmetic/1 -> Product1/1
  Ki/1 -> Shift Arithmetic/1
  Product2/1 -> 这个是缩小周期增益的/1
  Data Type Conversion3/1 -> Divide/2
  积分器运行频率/1 -> Data Type Conversion3/1

== system Senorless/FOC_PointModel/idq_Controller/PI Controller2/积分器//双边沿初始化/Reset_Block ==
  Xo : Inport
  Trigger : TriggerPort  TriggerType=either  VariantControl=(inherit)  OutputDataType=int8  InitialTriggerSignalState=zero  PortDimensions=1
  Data Store Write1 : DataStoreWrite  DataStoreName=tmp  IndexOptions=Index vector (dialog)  Indices=1  OutputSizes=1
  wires:
  Xo/1 -> Data Store Write1/1

== stateflow chart Senorless/FOC_PointModel/Chart ==
  state StopStage%出错暂停
    en:
    Motor_State = 0;
    Reset = 1;
    du:
    Motor_State = 0;
    Reset = 1;
    ex:
  state IDLE
    en:
    du:
    Motor_State = 0;
    Reset = 1;
    ex:
  state AlignStage%识别
    en:
    Reset = 0;
    Motor_State = 1;
    du:
    Motor_State = 1;
    ex:
  state CompStage%补偿
    en:
    Over_Curr_Cnt = 0;
    Motor_State = 3;
    du:
    Motor_State = 3;
    ex:
  state NSStage%辨识
    en:
    Motor_State = 2;
    du:
    Motor_State = 2;
    ex:
  state RunStage%闭环
    en:
    Motor_State = 4;
    du:
    Motor_State = 4;
    ex:
  state EndStage%出错结束
    en:
    Reset = 1;
    du:
    Reset = 1;
    ex:
  StopStage%出错暂停 -> IDLE : [after(200,msec)]
  AlignStage%识别 -> StopStage%出错暂停 [order 1] : [OverCurr_Err == 1]
  NSStage%辨识 -> StopStage%出错暂停 [order 1] : [OverCurr_Err == 1]
  CompStage%补偿 -> StopStage%出错暂停 [order 2] : [OverCurr_Err == 1]
  CompStage%补偿 -> StopStage%出错暂停 [order 1] : [after(500,msec)]
  (default) -> IDLE
  AlignStage%识别 -> NSStage%辨识 [order 2] : [after(50,msec)]
  NSStage%辨识 -> CompStage%补偿 [order 3] : [after(50,msec)]
  IDLE -> AlignStage%识别 : [Motor_OnOff ==1&& after(10,msec)]
  RunStage%闭环 -> EndStage%出错结束 [order 1] : [Run_Err == 1]
  CompStage%补偿 -> RunStage%闭环 [order 4] : [after(50,msec)]
  EndStage%出错结束 -> IDLE : [Motor_OnOff ==0]
  NSStage%辨识 -> IDLE [order 2] : [Motor_OnOff ==0]
  RunStage%闭环 -> IDLE [order 2] : [Motor_OnOff ==0]
  AlignStage%识别 -> IDLE [order 3] : [Motor_OnOff == 0]
  CompStage%补偿 -> IDLE [order 3] : [Motor_OnOff ==0 ]
  data: Motor_OnOff input int16; Reset output int16; Run_Err input boolean; OverCurr_Err input boolean; Over_Curr_Cnt local uint8 =0; Motor_State output uint8

== stateflow chart Senorless/FOC_PointModel/Observers/obs_chart ==
  state HFI_SMO2
    en,du:
    HFI_Output = bitshift(HFI_Input,-1);
    SMO_Output = SMO_Input;
  state HFI
    en,du:
    HFI_Output = HFI_Input;
    SMO_Output = [0;0];
  state HFI_SMO1
    en,du:
    HFI_Output = HFI_Input;
    SMO_Output = bitshift(SMO_Input,-1);
  state SMO
    en,du:
    HFI_Output = [0;0];
    SMO_Output = SMO_Input;
  state Begin
    en,du:
    HFI_Output = bitshift(HFI_Input,-1);
    SMO_Output = bitshift(SMO_Input,-1);
  HFI -> HFI_SMO2 : [Obs_Spd > OBS_SPD*2]
  HFI_SMO2 -> SMO : [after(10,msec)]
  HFI_SMO1 -> HFI : [after(10,msec)]
  SMO -> HFI_SMO1 : [Obs_Spd < OBS_SPD]
  Begin -> HFI [order 1] : [after(10,msec) && Obs_Spd < OBS_SPD]
  Begin -> SMO [order 2] : [after(10,msec) && Obs_Spd > OBS_SPD*2]
  (default) -> Begin
  data: SMO_Input input int32; SMO_Output output int32; HFI_Output output int32; HFI_Input input int32; Obs_Spd input int32 size=1; OBS_SPD parameter

== stateflow chart Senorless/FOC_PointModel/HF_Generator/Chart ==
  state ENABLE1
    en,du:
    output = boolean(1);
  state ENABLE
    en,du:
    output = boolean(1);
  state DISABLE
    en,du:
    output = boolean(0);
  (default) -> ENABLE
  ENABLE1 -> DISABLE : [after(50,msec)]
  ENABLE -> ENABLE1 : [Obs_SPD > (OBS_SPD*2 + OBS_SPD)]
  DISABLE -> ENABLE : [Obs_SPD<OBS_SPD*2]
  data: output output boolean; Obs_SPD input int32; OBS_SPD parameter

== stateflow chart Senorless/FOC_PointModel/观测器闭环//速度环/速度缓冲1 ==
  state SPD_Loop
    en:
    du:
    SPD_Ref = SPD_Loop;
    ex:
  state Open_Loop
    en:
    du:
    SPD_Ref = int32(SPD_MIN);
    ex:
  (default) -> Open_Loop
  Open_Loop -> SPD_Loop : [after(100,msec)]
  data: SPD_Ref output int32; SPD_Loop input int32; SPD_MIN parameter int32

== stateflow chart Senorless/FOC_PointModel/NS辨识/正负偏置 ==
  state Down
    en,du:
    output = int32(-comp);
  state Zero
    en,du:
    output = int32(0);
  state Up
    en,du:
    output = int32(comp);
  state Zero1
    en,du:
    output = int32(0);
  (default) -> Down
  Down -> Zero : [after(15,msec)]
  Up -> Zero1 : [after(15,msec)]
  Zero -> Up : [after(10,msec)]
  data: output output int32; comp input int32
